simulink model "LAB_TestConnections"  (R2020b)
settings: Solver=FixedStepDiscrete  StartTime=0.0  StopTime=10.0  FixedStep=0.01  RelTol=1e-3  EnableMultiTasking=on
libraries: BalRobTbx_baselib x5
settings Model: SILPILModeSetting=veronly  ExtModeTrigDuration=2  Creator=barondavid  LastModifiedBy=Musta
settings OptimizationCC: EnhancedBackFolding=on  PassReuseOutputArgsAs=Individual arguments  ZeroExternalMemoryAtStartup=off  ZeroInternalMemoryAtStartup=off  MaxStackSize=64  OptimizeBlockOrder=speed  DifferentSizesBufferReuse=on  OptimizationCustomize=off  EfficientTunableParamExpr=on
settings DebuggingCC: ParameterTunabilityLossMsg=error
settings HardwareCC: ProdBitPerInt=16  ProdBitPerPointer=16  ProdBitPerSizeT=16  ProdBitPerPtrDiffT=16  ProdLargestAtomicFloat=None  ProdWordSize=8  ProdHWDeviceType=Atmel->AVR
settings SFSimCC: MATLABDynamicMemAlloc=off
settings RTWCC: Description=Embedded Coder  SystemTargetFile=ert.tlc  HardwareBoard=Arduino Mega 2560  TemplateMakefile=ert_default_tmf  Toolchain=Arduino AVR  BuildConfiguration=Faster Runs
settings CodeAppCC: ForceParamTrailComments=on  IgnoreCustomStorageClasses=off  OperatorAnnotations=on  SimulinkDataObjDesc=on  SFDataObjDesc=on  InsertBlockDesc=on
settings ERTTargetCC: SupportContinuousTime=on  SupportVariableSizeSignals=on  ExtModeStaticAllocSize=2048

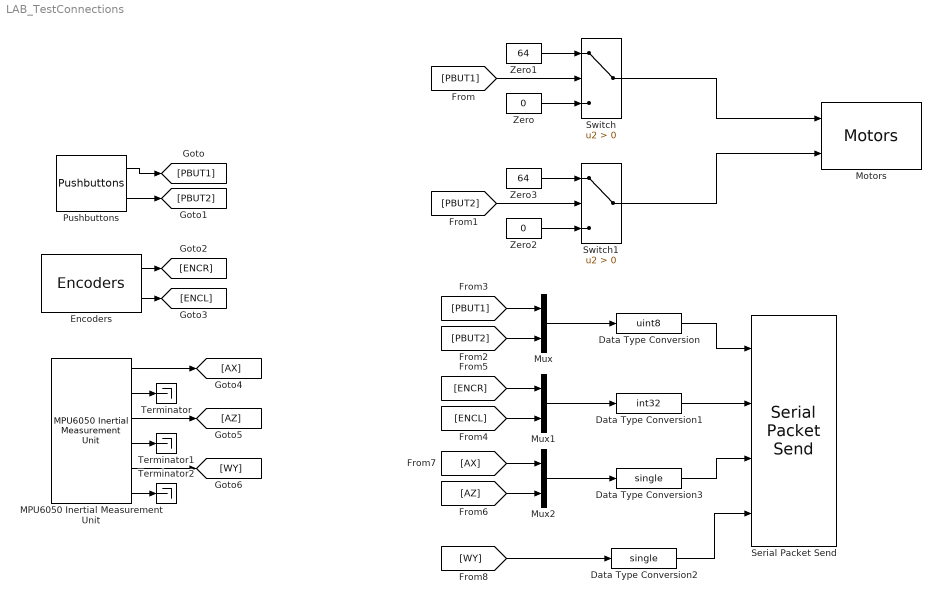
== system LAB_TestConnections ==
  Data Type Conversion : DataTypeConversion  OutDataTypeStr=uint8
  Data Type Conversion1 : DataTypeConversion  OutDataTypeStr=int32
  Data Type Conversion2 : DataTypeConversion  OutDataTypeStr=single
  Data Type Conversion3 : DataTypeConversion  OutDataTypeStr=single
  Encoders : BalRobTbx_baselib/Inputs/Encoders
      settings: SourceProductName=Balancing Robot Toolbox
  MPU6050 Inertial Measurement Unit : BalRobTbx_baselib/Inputs/MPU6050 Inertial Measurement Unit
      settings: SourceProductName=Balancing Robot Toolbox
  Motors : BalRobTbx_baselib/Outputs/Motors
      settings: SourceProductName=Balancing Robot Toolbox
  Mux : Mux  Inputs=2
  Mux1 : Mux  Inputs=2
  Mux2 : Mux  Inputs=2
  Pushbuttons : BalRobTbx_baselib/Inputs/Pushbuttons
      settings: SourceProductName=Balancing Robot Toolbox
  Serial Packet Send : BalRobTbx_baselib/Communication/Serial Packet Send  serialLinkOpt=Bluetooth  baudRateOpt=38400  waitHostTxCmd=on  txStartCmd=65  txStopCmd=66  packetSpec={'2*uint8','2*int32','2*single','single'}  cobsEncoded=on  nullTerminated=on  showEnablePort=off
      settings: SourceProductName=Balancing Robot Toolbox
  Switch : Switch  Criteria=u2 > Threshold
  Switch1 : Switch  Criteria=u2 > Threshold
  Terminator : Terminator
  Terminator1 : Terminator
  Terminator2 : Terminator
  Zero : Constant  Value=0  OutDataTypeStr=Inherit: Inherit via back propagation
  Zero1 : Constant  Value=64  OutDataTypeStr=Inherit: Inherit via back propagation
  Zero2 : Constant  Value=0  OutDataTypeStr=Inherit: Inherit via back propagation
  Zero3 : Constant  Value=64  OutDataTypeStr=Inherit: Inherit via back propagation
  wires:
  Mux/1 -> Data Type Conversion/1
  [PBUT2] -> Mux/2
  Mux2/1 -> Data Type Conversion3/1
  [PBUT1] -> Switch/2
  Zero3/1 -> Switch1/1
  Zero2/1 -> Switch1/3
  [WY] -> Data Type Conversion2/1
  Mux1/1 -> Data Type Conversion1/1
  Zero/1 -> Switch/3
  [ENCR] -> Mux1/1
  [AX] -> Mux2/1
  [PBUT1] -> Mux/1
  [ENCL] -> Mux1/2
  [PBUT2] -> Switch1/2
  Zero1/1 -> Switch/1
  [AZ] -> Mux2/2
  Data Type Conversion1/1 -> Serial Packet Send/2
  Data Type Conversion/1 -> Serial Packet Send/1
  Data Type Conversion3/1 -> Serial Packet Send/3
  Data Type Conversion2/1 -> Serial Packet Send/4
  Pushbuttons/1 -> [PBUT1]
  Pushbuttons/2 -> [PBUT2]
  Encoders/1 -> [ENCR]
  Encoders/2 -> [ENCL]
  MPU6050 Inertial Measurement Unit/6 -> Terminator2/1
  MPU6050 Inertial Measurement Unit/5 -> [WY]
  MPU6050 Inertial Measurement Unit/4 -> Terminator1/1
  MPU6050 Inertial Measurement Unit/3 -> [AZ]
  MPU6050 Inertial Measurement Unit/2 -> Terminator/1
  MPU6050 Inertial Measurement Unit/1 -> [AX]
  Switch1/1 -> Motors/2
  Switch/1 -> Motors/1
